simulink library "Driveline_FDiff"  (R2019b)
settings: Solver=VariableStepAuto  StartTime=0.0  StopTime=10.0  RelTol=1e-3
libraries: sm_car_lib x3, sm_lib x3, Driveshaft_ShaftsAll x2, fl_lib x1, sdl_lib x1
Description:
  | Component of Simscape Vehicle Templates Library
  | 
  | Copyright 2018-2020 The MathWorks, Inc.
settings Model: Creator=smiller  LastModifiedBy=smiller
settings DataIOCC: ReturnWorkspaceOutputs=off
settings DebuggingCC: ArithmeticOperatorsInVariantConditions=warning
settings SFSimCC: CustomCodeUndefinedFunction=UseInterfaceOnly

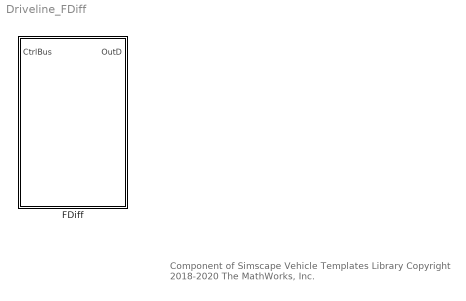
== system Driveline_FDiff ==
  note: Component of Simscape Vehicle Templates Library
      | Copyright 2018-2020 The MathWorks, Inc.
  FDiff : Subsystem  Tag=PublishSubsystem  VariantControl=IndepFRDiffFDiffR  mask(Driveline, Front Differential){InitTriggerDropdown=0}
      mask prompts: InitTriggerDropdown "Initialization Trigger Dropdown"
      mask help: Models front axle with differential.
      mask init:
      | curblk = gcb;
      | 
      | % Trigger Mask Initialization for 
      | % variant subsystems below this level
      | sm_car_lib_maskInitTrigger(curblk)
      mask TypeOptions InitTriggerDropdown: 0 | 1
      mask Display: image('sm_car_vehicle_driveline_fdiff_IMAGE.png');

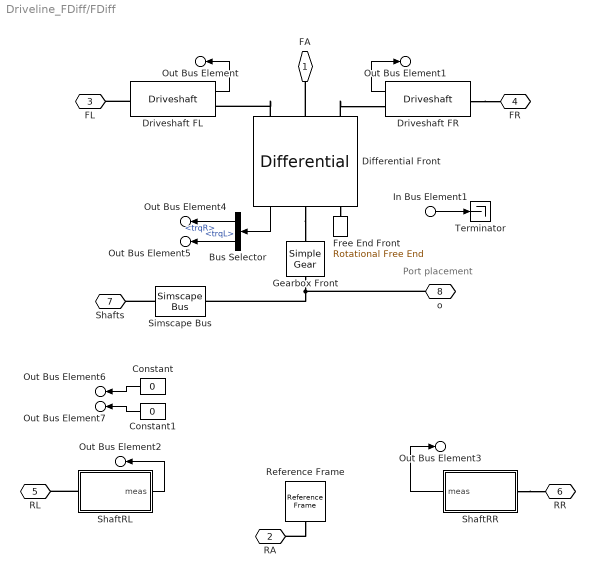
== system Driveline_FDiff/FDiff ==
  note: Port
      | placement
  In Bus Element1 : Inport  PortName=CtrlBus
  Bus Selector : BusSelector  OutputSignals=trqR,trqL
  Constant : Constant  Value=0
  Constant1 : Constant  Value=0
  Differential Front : sm_car_lib/Driveline/Differential  VariantControl=Variant1  Differential=Driveline.DifferentialF  VariantLabel=Driveline.DifferentialF.class.Value  InitTriggerDropdown=0
      settings: AttributesFormatString=%<ActiveVariant>
  Driveshaft FL : sm_car_lib/Driveline/Driveshaft  VariantControl=Variant1  popup_leftRight=Left  Driveshaft=Driveline.DriveshaftFL  VariantLabel=Driveline.DriveshaftFL.class.Value  InitTriggerDropdown=0
      settings: AttributesFormatString=%<ActiveVariant>
  Driveshaft FR : sm_car_lib/Driveline/Driveshaft  VariantControl=Variant1  popup_leftRight=Right  Driveshaft=Driveline.DriveshaftFR  VariantLabel=Driveline.DriveshaftFR.class.Value  InitTriggerDropdown=0
      settings: AttributesFormatString=%<ActiveVariant>
  Free End Front : fl_lib/Mechanical/Rotational Elements/Rotational Free End  w_specify=off  w_priority=None  w=0 rad/s  w_nominal_specify=off  w_nominal_unit=rad/s  w_nominal_value=1
      settings: SourceProductName=Simscape  SourceProductBaseCode=SS
  Gearbox Front : sdl_lib/Gears/Simple Gear  ratio=Driveline.GearboxF.ratio.Value  rotation_direction=1  friction_model=1  T_noload=0.1 N*m  T_nom=5 N*m  efficiency_nom=0.8  efficiency=0.8  mu_visc=[0, 0] N*m/(rad/s)  w_thr=0.01 rad/s  pwr_thr=0.001 W  enable_faults=0  efficiency_fault=0.05  external_fault=simscape.enum.onoff.off  temporal_fault=0  fault_time=5 s  fault_angles=pi / 12 rad  report_fault=1  temperature_TLU=[280, 300, 320] K  load_TLU=[1, 5, 10] N*m  efficiency_TLU=[.95, .9, .85]  efficiency_TLU2=[.85, .8, .75; .95, .9, .85; .85, .8, .7]  thermal_mass=50 J/K  T_init=300 K
      settings: SourceProductName=Simscape Driveline
  Reference Frame : sm_lib/Frames and Transforms/Reference Frame
  ShaftRL : Subsystem  VariantControl=Shaft1D  mask(Driveshaft Assembly (1D)){}
      mask help: Models a shaft as a 1D mechanical connection.
  ShaftRR : Subsystem  VariantControl=Shaft1D  mask(Driveshaft Assembly (1D)){}
      mask help: Models a shaft as a 1D mechanical connection.
  Simscape Bus : SimscapeBus  HierarchyStrings=ShaftF
  Terminator : Terminator
  FA : PMIOPort  Side=Left
  RA : PMIOPort  Port=2  Side=Right
  FL : PMIOPort  Port=3  Side=Left
  FR : PMIOPort  Port=4  Side=Right
  RL : PMIOPort  Port=5  Side=Left
  RR : PMIOPort  Port=6  Side=Right
  Shafts : PMIOPort  Port=7  Side=Left
  o : PMIOPort  Port=8  Side=Right
  Out Bus Element6 : Outport  VectorParamsAs1DForOutWhenUnconnected=off  PortName=OutD  Element=MDriveshaftRL
  Out Bus Element7 : Outport  VectorParamsAs1DForOutWhenUnconnected=off  PortName=OutD  Element=MDriveshaftRR
  Out Bus Element4 : Outport  VectorParamsAs1DForOutWhenUnconnected=off  PortName=OutD  Element=MDriveshaftFL
  Out Bus Element5 : Outport  VectorParamsAs1DForOutWhenUnconnected=off  PortName=OutD  Element=MDriveshaftFR
  Out Bus Element : Outport  VectorParamsAs1DForOutWhenUnconnected=off  PortName=OutD  Element=anDriveshaftFL
  Out Bus Element1 : Outport  VectorParamsAs1DForOutWhenUnconnected=off  PortName=OutD  Element=anDriveshaftFR
  Out Bus Element2 : Outport  VectorParamsAs1DForOutWhenUnconnected=off  PortName=OutD  Element=anDriveshaftRL
  Out Bus Element3 : Outport  VectorParamsAs1DForOutWhenUnconnected=off  PortName=OutD  Element=anDriveshaftRR
  wires:
  In Bus Element1/1 -> Terminator/1
  Bus Selector/2 -> Out Bus Element5/1  "<trqL>"
  Bus Selector/1 -> Out Bus Element4/1  "<trqR>"
  Constant/1 -> Out Bus Element6/1
  Constant1/1 -> Out Bus Element7/1
  Differential Front/1 -> Bus Selector/1
  ShaftRR/1(meas) -> Out Bus Element3/1
  ShaftRL/1(meas) -> Out Bus Element2/1
  Driveshaft FL/1 -> Out Bus Element/1
  Driveshaft FR/1 -> Out Bus Element1/1
  connections:
  Simscape Bus/RConn1 -- Shafts/RConn1
  ShaftRL/LConn1 -- RL/RConn1
  ShaftRR/LConn1 -- RR/RConn1
  Differential Front/RConn1 -- Gearbox Front/RConn1
  Reference Frame/RConn1 -- RA/RConn1
  Differential Front/LConn2 -- FA/RConn1
  Driveshaft FL/LConn1 -- FL/RConn1
  Driveshaft FR/LConn1 -- FR/RConn1
  Differential Front/LConn3 -- Driveshaft FR/RConn1
  Differential Front/LConn1 -- Driveshaft FL/RConn1
  Differential Front/RConn2 -- Free End Front/LConn1
  Gearbox Front/LConn1 -- o/RConn1 -- Simscape Bus/LConn1

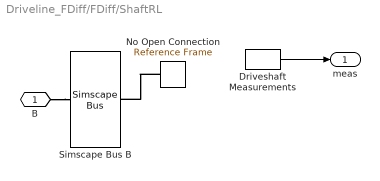
== system Driveline_FDiff/FDiff/ShaftRL ==
  Driveshaft Measurements : Driveshaft_ShaftsAll/Driveshaft Measurements  SystemSampleTime=-1  Latency=0  AutoFrameSizeCalculation=off
  No Open Connection : sm_lib/Frames and Transforms/Reference Frame
  Simscape Bus B : SimscapeBus  HierarchyStrings=AxleIn
  B : PMIOPort  Side=Left
  meas : Outport  VectorParamsAs1DForOutWhenUnconnected=off
  wires:
  Driveshaft Measurements/1 -> meas/1
  connections:
  B/RConn1 -- Simscape Bus B/RConn1
  No Open Connection/RConn1 -- Simscape Bus B/LConn1

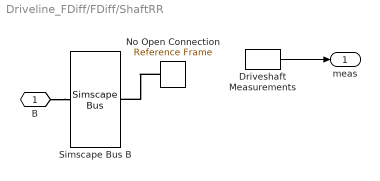
== system Driveline_FDiff/FDiff/ShaftRR ==
  Driveshaft Measurements : Driveshaft_ShaftsAll/Driveshaft Measurements  SystemSampleTime=-1  Latency=0  AutoFrameSizeCalculation=off
  No Open Connection : sm_lib/Frames and Transforms/Reference Frame
  Simscape Bus B : SimscapeBus  HierarchyStrings=AxleIn
  B : PMIOPort  Side=Left
  meas : Outport  VectorParamsAs1DForOutWhenUnconnected=off
  wires:
  Driveshaft Measurements/1 -> meas/1
  connections:
  B/RConn1 -- Simscape Bus B/RConn1
  No Open Connection/RConn1 -- Simscape Bus B/LConn1
